simulink model "ForwardKinematic_YuMi"  (R2024a)
settings: Solver=VariableStepAuto  StartTime=0.0  StopTime=inf  RelTol=1e-3
PreLoadFcn:
  | Yumirobot = loadrobot("abbYuMi");
  | assignin('base', 'Yumirobot', Yumirobot);
InitFcn:
  | Yumirobot = loadrobot("abbYuMi");
  | assignin('base', 'Yumirobot', Yumirobot);
(part 1 of 23)
settings Model: Creator=Alushi  LastModifiedBy=LYA31

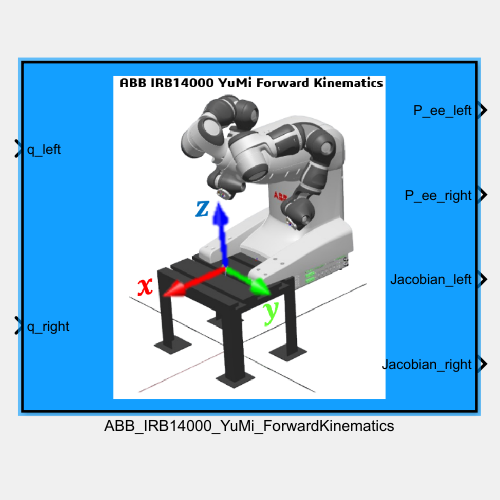
[thumbnail: Simulink's stored preview of the top-level diagram]
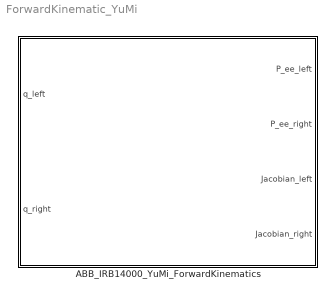
== system ForwardKinematic_YuMi ==
  ABB_IRB14000_YuMi_ForwardKinematics : MATLAB Function  TreatAsAtomicUnit=on
